simulink model "Energy_Storage_System"  (R2022b)
settings: Solver=FixedStepAuto  StartTime=0.0  StopTime=20000  FixedStep=1  RelTol=1e-3
model workspace (MAT data in the model file):
  C_space = 0.4
  Dilate = 0.1
  P0 = 100
  P_in_comp = 100
  T0 = 310
  T_coldwater_in = 293
  T_coldwater_out = 353
  T_in_comp = 300
  V_compress = 0.1
  V_storage = 310000
  Y_abhot = 1.295
  m0 = 320000
  rotor_speed = 80
settings Model: Creator=Crapon  LastModifiedBy=Crapon

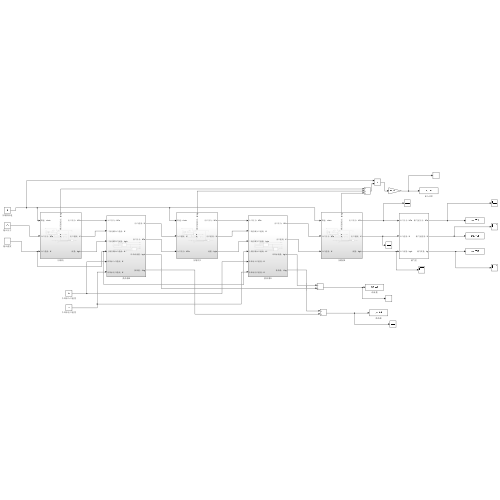
[thumbnail: Simulink's stored preview of the top-level diagram]
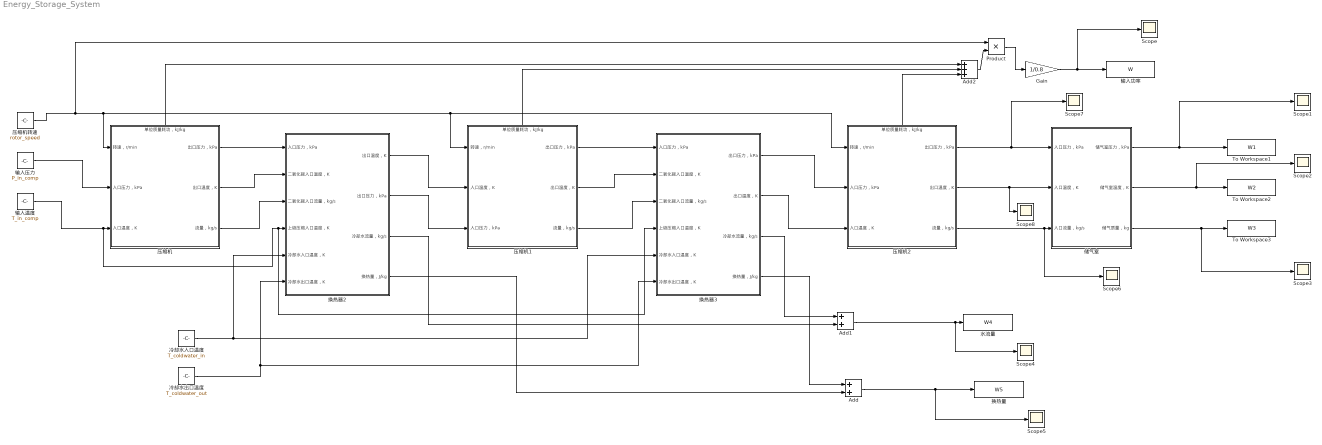
== system Energy_Storage_System ==
  Add : Sum
  Add1 : Sum
  Add2 : Sum  Inputs=+++
  Gain : Gain  Gain=1/0.8
  Product : Product
  Scope{,1..8} (9 alike) : Scope
  To Workspace1 : ToWorkspace  VariableName=W1  SaveFormat=Timeseries  SampleTime=-1
  To Workspace2 : ToWorkspace  VariableName=W2  SaveFormat=Timeseries  SampleTime=-1
  To Workspace3 : ToWorkspace  VariableName=W3  SaveFormat=Timeseries  SampleTime=-1
  储气室 : Subsystem
  冷却水入口温度 : Constant  Value=T_coldwater_in
  冷却水出口温度 : Constant  Value=T_coldwater_out
  压缩机 : Subsystem
      settings: PortSchema="{\"entries\":[{\"content\":{\"sides\":[{\"content\":{\"connectorIds\":[\"In1\",\"In2\",\"In3\"]},\"type\":\"ConnectorPlacement.EquallySpacedRectSide\",\"uuid\":\"17bf042e-cadd-48a6-8dfd-0be3cb7c0c8b\"},{\"content\":{\"connectorIds\":[\"Out1\",\"Out2\",\"Out3\"],\"side\":\"RIGHT\"},\"type\":\"ConnectorPlacement.EquallySpacedRectSide\",\"uuid\":\"9580532f-fe29-4788-9d7a-ca1c4a6711f8\"},{\"content\":{\"connectorIds\":[\"Out4\"],\"side\":\"TOP\"},\"type\":\"ConnectorPlacement.EquallySpacedRectSide\",\"uuid\":\"3a849305-9831-4dda-bb31-32b1caf0413e\"}]},\"type\":\"ConnectorPlacement.EquallySpacedConnector\",\"uuid\":\"fce5bf21-7d26-4726-80d8-4928c417d458\"}],\"packageUris\":[\"http://schema.mathworks.com/mf0/Connector/R2020b\"],\"version\":\"1.0\"}"
  压缩机1 : Subsystem
      settings: PortSchema="{\"entries\":[{\"content\":{\"sides\":[{\"content\":{\"connectorIds\":[\"In1\",\"In2\",\"In3\"]},\"type\":\"ConnectorPlacement.EquallySpacedRectSide\",\"uuid\":\"17bf042e-cadd-48a6-8dfd-0be3cb7c0c8b\"},{\"content\":{\"connectorIds\":[\"Out1\",\"Out2\",\"Out3\"],\"side\":\"RIGHT\"},\"type\":\"ConnectorPlacement.EquallySpacedRectSide\",\"uuid\":\"9580532f-fe29-4788-9d7a-ca1c4a6711f8\"},{\"content\":{\"connectorIds\":[\"Out4\"],\"side\":\"TOP\"},\"type\":\"ConnectorPlacement.EquallySpacedRectSide\",\"uuid\":\"3a849305-9831-4dda-bb31-32b1caf0413e\"}]},\"type\":\"ConnectorPlacement.EquallySpacedConnector\",\"uuid\":\"fce5bf21-7d26-4726-80d8-4928c417d458\"}],\"packageUris\":[\"http://schema.mathworks.com/mf0/Connector/R2020b\"],\"version\":\"1.0\"}"
  压缩机2 : Subsystem
      settings: PortSchema="{\"entries\":[{\"content\":{\"sides\":[{\"content\":{\"connectorIds\":[\"In1\",\"In2\",\"In3\"]},\"type\":\"ConnectorPlacement.EquallySpacedRectSide\",\"uuid\":\"17bf042e-cadd-48a6-8dfd-0be3cb7c0c8b\"},{\"content\":{\"connectorIds\":[\"Out1\",\"Out2\",\"Out3\"],\"side\":\"RIGHT\"},\"type\":\"ConnectorPlacement.EquallySpacedRectSide\",\"uuid\":\"9580532f-fe29-4788-9d7a-ca1c4a6711f8\"},{\"content\":{\"connectorIds\":[\"Out4\"],\"side\":\"TOP\"},\"type\":\"ConnectorPlacement.EquallySpacedRectSide\",\"uuid\":\"3a849305-9831-4dda-bb31-32b1caf0413e\"}]},\"type\":\"ConnectorPlacement.EquallySpacedConnector\",\"uuid\":\"fce5bf21-7d26-4726-80d8-4928c417d458\"}],\"packageUris\":[\"http://schema.mathworks.com/mf0/Connector/R2020b\"],\"version\":\"1.0\"}"
  压缩机转速 : Constant  Value=rotor_speed
  换热器2 : Subsystem
  换热器3 : Subsystem
  换热量 : ToWorkspace  VariableName=W5  SaveFormat=Timeseries  SampleTime=-1
  水流量 : ToWorkspace  VariableName=W4  SaveFormat=Timeseries  SampleTime=-1
  输入功率 : ToWorkspace  VariableName=W  SaveFormat=Timeseries  SampleTime=-1
  输入压力 : Constant  Value=P_in_comp
  输入温度 : Constant  Value=T_in_comp
  wires:
  压缩机/1(出口压力，kPa) -> 换热器2/1(入口压力，kPa)
  压缩机/2(出口温度，K) -> 换热器2/2(二氧化碳入口温度，K)
  压缩机/3(流量，kg/s) -> 换热器2/3(二氧化碳入口流量，kg/s)
  输入压力/1 -> 压缩机/2(入口压力，kPa)
  输入温度/1 -> 换热器3/4(上级压缩入口温度，K), 换热器2/4(上级压缩入口温度，K), 压缩机/3(入口温度，K)
  压缩机转速/1 -> Product/1, 压缩机/1(转速，r/min), 压缩机1/1(转速，r/min), 压缩机2/1(转速，r/min)
  压缩机1/1(出口压力，kPa) -> 换热器3/1(入口压力，kPa)
  压缩机1/2(出口温度，K) -> 换热器3/2(二氧化碳入口温度，K)
  压缩机1/3(流量，kg/s) -> 换热器3/3(二氧化碳入口流量，kg/s)
  换热器3/1(出口压力，kPa) -> 压缩机2/2(入口压力，kPa)
  换热器3/2(出口温度，K) -> 压缩机2/3(入口温度，K)
  压缩机2/1(出口压力，kPa) -> Scope7/1, 储气室/1(入口压力，kPa)
  压缩机2/2(出口温度，K) -> Scope8/1, 储气室/2(入口温度，K)
  压缩机2/3(流量，kg/s) -> Scope6/1, 储气室/3(入口流量，kg/s)
  换热器2/4(换热量，J/kg) -> Add/2
  换热器3/4(换热量，J/kg) -> Add/1
  换热器2/3(冷却水流量，kg/s) -> Add1/2
  换热器3/3(冷却水流量，kg/s) -> Add1/1
  压缩机/4(单位质量耗功，kJ/kg) -> Add2/1
  压缩机1/4(单位质量耗功，kJ/kg) -> Add2/2
  压缩机2/4(单位质量耗功，kJ/kg) -> Add2/3
  Gain/1 -> Scope/1, 输入功率/1
  储气室/1(储气室压力，kPa) -> To Workspace1/1, Scope1/1
  储气室/2(储气室温度，K) -> To Workspace2/1, Scope2/1
  储气室/3(储气质量，kg) -> Scope3/1, To Workspace3/1
  Add1/1 -> Scope4/1, 水流量/1
  Add/1 -> Scope5/1, 换热量/1
  冷却水入口温度/1 -> 换热器2/5(冷却水入口温度，K), 换热器3/5(冷却水入口温度，K)
  冷却水出口温度/1 -> 换热器3/6(冷却水出口温度，K), 换热器2/6(冷却水出口温度，K)
  换热器2/2(出口压力，kPa) -> 压缩机1/3(入口压力，kPa)
  换热器2/1(出口温度，K) -> 压缩机1/2(入口温度，K)
  Add2/1 -> Product/2
  Product/1 -> Gain/1

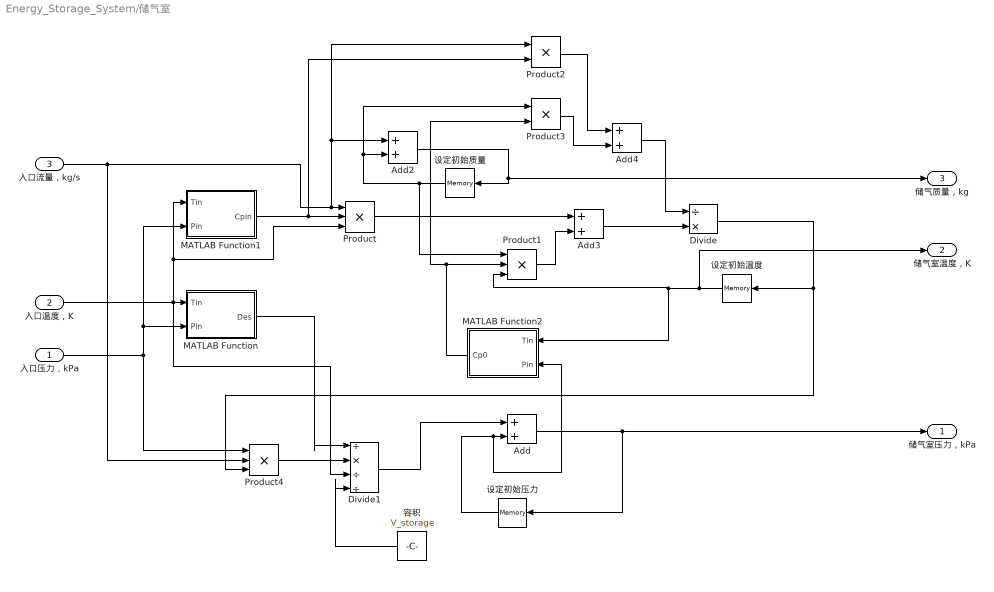
== system Energy_Storage_System/储气室 ==
  入口压力，kPa : Inport
  入口温度，K : Inport  Port=2
  入口流量，kg/s : Inport  Port=3
  Add{,2..4} (4 alike) : Sum
  Divide : Product  Inputs=/*
  Divide1 : Product  Inputs=/*//
  MATLAB Function : MATLAB Function  TreatAsAtomicUnit=on
  MATLAB Function1 : MATLAB Function  TreatAsAtomicUnit=on
  MATLAB Function2 : MATLAB Function  TreatAsAtomicUnit=on
  Product : Product  Inputs=3
  Product1 : Product  Inputs=3
  Product2 : Product
  Product3 : Product
  Product4 : Product  Inputs=3
  容积 : Constant  Value=V_storage
  设定初始压力 : Memory  InitialCondition=P0
  设定初始温度 : Memory  InitialCondition=T0
  设定初始质量 : Memory  InitialCondition=m0
  储气室压力，kPa : Outport
  储气室温度，K : Outport  Port=2
  储气质量，kg : Outport  Port=3
  wires:
  入口流量，kg/s/1 -> Product4/2, Product2/1, Add2/1, Product/1
  设定初始质量/1 -> Product1/1, Product3/1, Add2/2
  Product2/1 -> Add4/1
  MATLAB Function1/1(Cpin) -> Product/2, Product2/2
  Product4/1 -> Divide1/2
  MATLAB Function2/1(Cp0) -> Product1/2, Product3/2
  Divide1/1 -> Add/1
  入口温度，K/1 -> MATLAB Function1/1(Tin), Product/3, MATLAB Function/1(Tin), Divide1/3
  Product1/1 -> Add3/2
  Add/1 -> 储气室压力，kPa/1, 设定初始压力/1
  入口压力，kPa/1 -> Product4/1, MATLAB Function1/2(Pin), MATLAB Function/2(Pin)
  Add4/1 -> Divide/1
  设定初始压力/1 -> MATLAB Function2/2(Pin), Add/2
  容积/1 -> Divide1/4
  Product3/1 -> Add4/2
  MATLAB Function/1(Des) -> Divide1/1
  Add3/1 -> Divide/2
  Product/1 -> Add3/1
  Divide/1 -> Product4/3, 设定初始温度/1
  Add2/1 -> 设定初始质量/1, 储气质量，kg/1
  设定初始温度/1 -> 储气室温度，K/1, MATLAB Function2/1(Tin), Product1/3

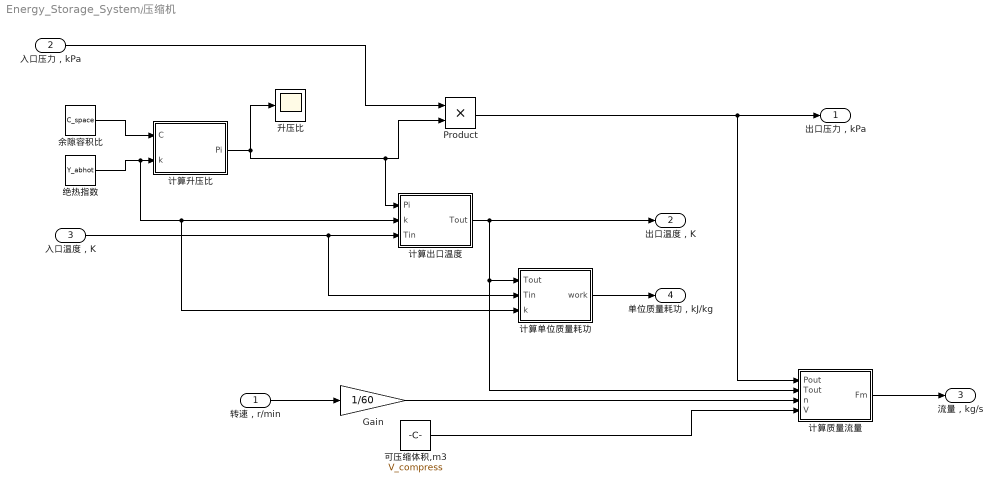
== system Energy_Storage_System/压缩机 ==
  转速，r/min : Inport
  入口压力，kPa : Inport  Port=2
  入口温度，K : Inport  Port=3
  Gain : Gain  Gain=1/60
  Product : Product
  余隙容积比 : Constant  Value=C_space
  升压比 : Scope
  可压缩体积,m3 : Constant  Value=V_compress
  绝热指数 : Constant  Value=Y_abhot
  计算出口温度 : MATLAB Function  TreatAsAtomicUnit=on
  计算升压比 : MATLAB Function  TreatAsAtomicUnit=on
  计算单位质量耗功 : MATLAB Function  TreatAsAtomicUnit=on
  计算质量流量 : MATLAB Function  TreatAsAtomicUnit=on
  出口压力，kPa : Outport
  出口温度，K : Outport  Port=2
  流量，kg/s : Outport  Port=3
  单位质量耗功，kJ/kg : Outport  Port=4
  wires:
  余隙容积比/1 -> 计算升压比/1(C)
  入口压力，kPa/1 -> Product/1
  绝热指数/1 -> 计算单位质量耗功/3(k), 计算出口温度/2(k), 计算升压比/2(k)
  Product/1 -> 计算质量流量/1(Pout), 出口压力，kPa/1
  计算单位质量耗功/1(work) -> 单位质量耗功，kJ/kg/1
  计算升压比/1(Pi) -> 计算出口温度/1(Pi), Product/2, 升压比/1
  入口温度，K/1 -> 计算单位质量耗功/2(Tin), 计算出口温度/3(Tin)
  计算出口温度/1(Tout) -> 出口温度，K/1, 计算质量流量/2(Tout), 计算单位质量耗功/1(Tout)
  计算质量流量/1(Fm) -> 流量，kg/s/1
  转速，r/min/1 -> Gain/1
  Gain/1 -> 计算质量流量/3(n)
  可压缩体积,m3/1 -> 计算质量流量/4(V)

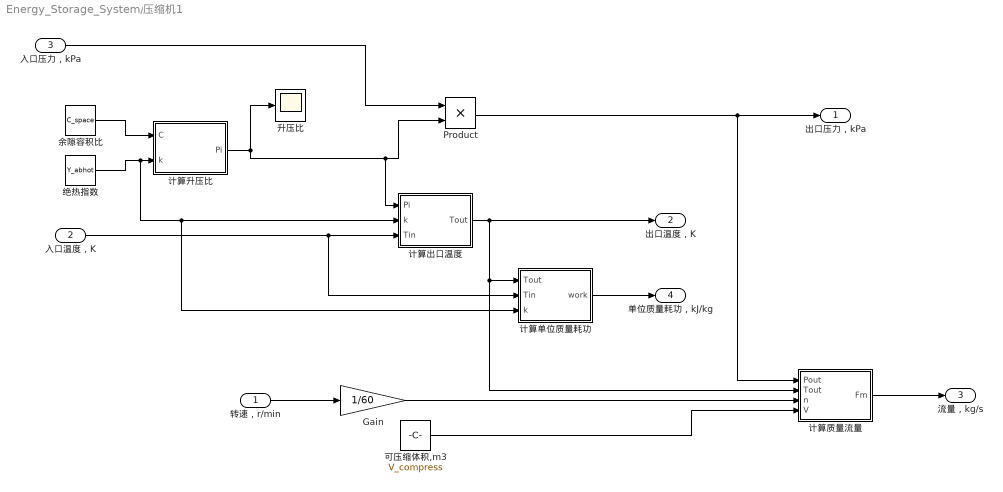
== system Energy_Storage_System/压缩机1 ==
  转速，r/min : Inport
  入口温度，K : Inport  Port=2
  入口压力，kPa : Inport  Port=3
  Gain : Gain  Gain=1/60
  Product : Product
  余隙容积比 : Constant  Value=C_space
  升压比 : Scope
  可压缩体积,m3 : Constant  Value=V_compress
  绝热指数 : Constant  Value=Y_abhot
  计算出口温度 : MATLAB Function  TreatAsAtomicUnit=on
  计算升压比 : MATLAB Function  TreatAsAtomicUnit=on
  计算单位质量耗功 : MATLAB Function  TreatAsAtomicUnit=on
  计算质量流量 : MATLAB Function  TreatAsAtomicUnit=on
  出口压力，kPa : Outport
  出口温度，K : Outport  Port=2
  流量，kg/s : Outport  Port=3
  单位质量耗功，kJ/kg : Outport  Port=4
  wires:
  可压缩体积,m3/1 -> 计算质量流量/4(V)
  Gain/1 -> 计算质量流量/3(n)
  转速，r/min/1 -> Gain/1
  计算质量流量/1(Fm) -> 流量，kg/s/1
  计算出口温度/1(Tout) -> 计算单位质量耗功/1(Tout), 计算质量流量/2(Tout), 出口温度，K/1
  入口温度，K/1 -> 计算出口温度/3(Tin), 计算单位质量耗功/2(Tin)
  计算升压比/1(Pi) -> 升压比/1, Product/2, 计算出口温度/1(Pi)
  计算单位质量耗功/1(work) -> 单位质量耗功，kJ/kg/1
  Product/1 -> 出口压力，kPa/1, 计算质量流量/1(Pout)
  绝热指数/1 -> 计算升压比/2(k), 计算出口温度/2(k), 计算单位质量耗功/3(k)
  入口压力，kPa/1 -> Product/1
  余隙容积比/1 -> 计算升压比/1(C)

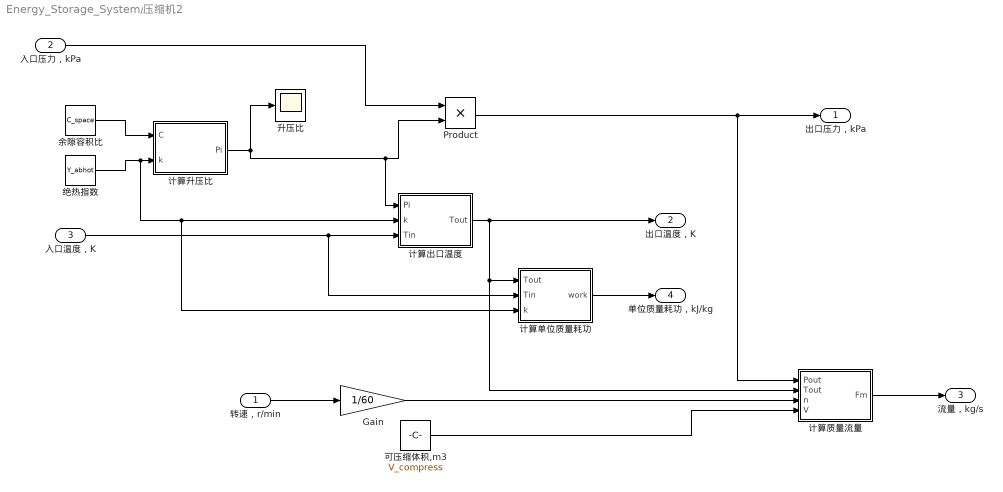
== system Energy_Storage_System/压缩机2 ==
  转速，r/min : Inport
  入口压力，kPa : Inport  Port=2
  入口温度，K : Inport  Port=3
  Gain : Gain  Gain=1/60
  Product : Product
  余隙容积比 : Constant  Value=C_space
  升压比 : Scope
  可压缩体积,m3 : Constant  Value=V_compress
  绝热指数 : Constant  Value=Y_abhot
  计算出口温度 : MATLAB Function  TreatAsAtomicUnit=on
  计算升压比 : MATLAB Function  TreatAsAtomicUnit=on
  计算单位质量耗功 : MATLAB Function  TreatAsAtomicUnit=on
  计算质量流量 : MATLAB Function  TreatAsAtomicUnit=on
  出口压力，kPa : Outport
  出口温度，K : Outport  Port=2
  流量，kg/s : Outport  Port=3
  单位质量耗功，kJ/kg : Outport  Port=4
  wires:
  余隙容积比/1 -> 计算升压比/1(C)
  入口压力，kPa/1 -> Product/1
  绝热指数/1 -> 计算单位质量耗功/3(k), 计算出口温度/2(k), 计算升压比/2(k)
  Product/1 -> 计算质量流量/1(Pout), 出口压力，kPa/1
  计算单位质量耗功/1(work) -> 单位质量耗功，kJ/kg/1
  计算升压比/1(Pi) -> 计算出口温度/1(Pi), Product/2, 升压比/1
  入口温度，K/1 -> 计算单位质量耗功/2(Tin), 计算出口温度/3(Tin)
  计算出口温度/1(Tout) -> 出口温度，K/1, 计算质量流量/2(Tout), 计算单位质量耗功/1(Tout)
  计算质量流量/1(Fm) -> 流量，kg/s/1
  转速，r/min/1 -> Gain/1
  Gain/1 -> 计算质量流量/3(n)
  可压缩体积,m3/1 -> 计算质量流量/4(V)

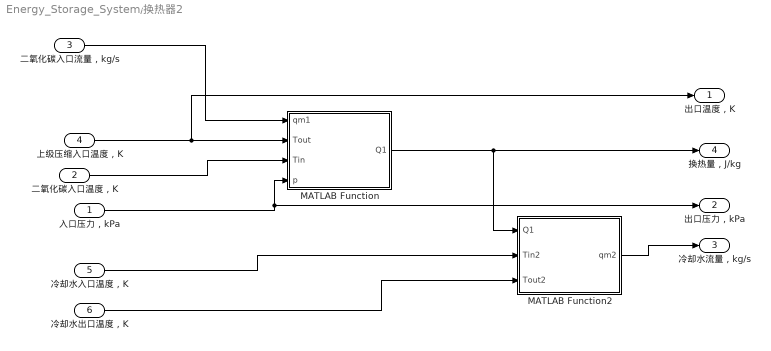
== system Energy_Storage_System/换热器2 ==
  入口压力，kPa : Inport
  二氧化碳入口温度，K : Inport  Port=2
  二氧化碳入口流量，kg/s : Inport  Port=3
  上级压缩入口温度，K : Inport  Port=4
  冷却水入口温度，K : Inport  Port=5
  冷却水出口温度，K : Inport  Port=6
  MATLAB Function : MATLAB Function  TreatAsAtomicUnit=on
  MATLAB Function2 : MATLAB Function  TreatAsAtomicUnit=on
  出口温度，K : Outport
  出口压力，kPa : Outport  Port=2
  冷却水流量，kg/s : Outport  Port=3
  换热量，J/kg : Outport  Port=4
  wires:
  入口压力，kPa/1 -> 出口压力，kPa/1, MATLAB Function/4(p)
  二氧化碳入口流量，kg/s/1 -> MATLAB Function/1(qm1)
  上级压缩入口温度，K/1 -> MATLAB Function/2(Tout), 出口温度，K/1
  二氧化碳入口温度，K/1 -> MATLAB Function/3(Tin)
  MATLAB Function2/1(qm2) -> 冷却水流量，kg/s/1
  冷却水入口温度，K/1 -> MATLAB Function2/2(Tin2)
  冷却水出口温度，K/1 -> MATLAB Function2/3(Tout2)
  MATLAB Function/1(Q1) -> MATLAB Function2/1(Q1), 换热量，J/kg/1

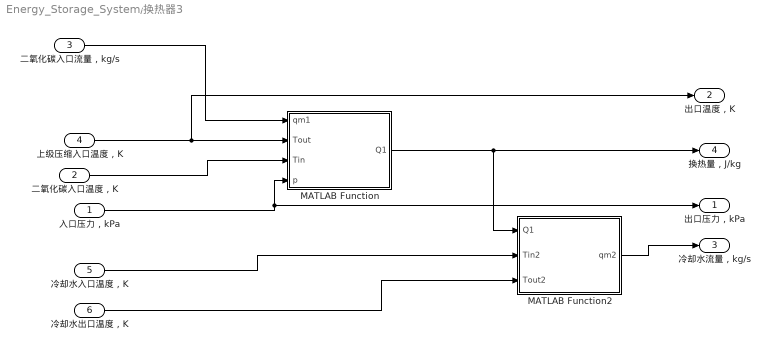
== system Energy_Storage_System/换热器3 ==
  入口压力，kPa : Inport
  二氧化碳入口温度，K : Inport  Port=2
  二氧化碳入口流量，kg/s : Inport  Port=3
  上级压缩入口温度，K : Inport  Port=4
  冷却水入口温度，K : Inport  Port=5
  冷却水出口温度，K : Inport  Port=6
  MATLAB Function : MATLAB Function  TreatAsAtomicUnit=on
  MATLAB Function2 : MATLAB Function  TreatAsAtomicUnit=on
  出口压力，kPa : Outport
  出口温度，K : Outport  Port=2
  冷却水流量，kg/s : Outport  Port=3
  换热量，J/kg : Outport  Port=4
  wires:
  MATLAB Function/1(Q1) -> 换热量，J/kg/1, MATLAB Function2/1(Q1)
  冷却水出口温度，K/1 -> MATLAB Function2/3(Tout2)
  冷却水入口温度，K/1 -> MATLAB Function2/2(Tin2)
  MATLAB Function2/1(qm2) -> 冷却水流量，kg/s/1
  二氧化碳入口温度，K/1 -> MATLAB Function/3(Tin)
  上级压缩入口温度，K/1 -> 出口温度，K/1, MATLAB Function/2(Tout)
  二氧化碳入口流量，kg/s/1 -> MATLAB Function/1(qm1)
  入口压力，kPa/1 -> MATLAB Function/4(p), 出口压力，kPa/1

== matlab function Energy_Storage_System/压缩机2/计算出口温度 ==
  data: Pi input; Tout output; k input; Tin input
function Tout= fcn(Pi, k, Tin)

Tout=Tin*(Pi)^((k-1)/k);

== matlab function Energy_Storage_System/储气室/MATLAB Function1 ==
  data: Tin input; Cpin output; Pin input
function Cpin = fcn(Tin,Pin)
coder.extrinsic('refpropm');
Cpin=zeros(1);
Cpin = refpropm('C','T',Tin,'P',Pin,'CO2');

== matlab function Energy_Storage_System/压缩机2/计算升压比 ==
  data: C input; Pi output; k input
function Pi = fcn(C, k)

Pi =(1+1/C)^k;

== matlab function Energy_Storage_System/压缩机2/计算单位质量耗功 ==
  data: Tout input; Tin input; k input; work output
function work= fcn(Tout,Tin,k)
Rg=0.189;
work=(k/(k-1))*Rg*(Tout-Tin);

== matlab function Energy_Storage_System/压缩机2/计算质量流量 ==
  data: Pout input; Tout input; n input; V input; Fm output
function Fm = fcn(Pout, Tout,n, V)
coder.extrinsic('refpropm');
a=zeros(1);
a=refpropm('D','T',Tout,'P',Pout,'CO2');
Fm = a*V*n;

== matlab function Energy_Storage_System/换热器2/MATLAB Function ==
  data: qm1 input; Tout input; Tin input; Q1 output; p input
function Q1 = fc(qm1,Tout,Tin,p)
coder.extrinsic('refpropm');
cp=zeros(1);
t=(Tin+Tout)/2;
cp=refpropm('C','T',t,'P',p,'CO2');
Q1= qm1*cp*(Tout-Tin);

== matlab function Energy_Storage_System/换热器2/MATLAB Function2 ==
  data: Q1 input; Tin2 input; Tout2 input; qm2 output
function qm2 = fcn(Q1,Tin2,Tout2)
coder.extrinsic('refpropm');
cp=zeros(1);
t=(Tin2+Tout2)/2;
cp=refpropm('C','T',t,'Q',0,'water');
qm2= Q1/(cp*(Tout2-Tin2));

== matlab function Energy_Storage_System/换热器3/MATLAB Function ==
  data: qm1 input; Tout input; Tin input; Q1 output; p input
function Q1 = fc(qm1,Tout,Tin,p)
coder.extrinsic('refpropm');
t=(Tin+Tout)/2;
cp=zeros(1);
cp=refpropm('C','T',t,'P',p,'CO2');
Q1= qm1*cp*(Tout-Tin);

== matlab function Energy_Storage_System/换热器3/MATLAB Function2 ==
  data: Q1 input; Tin2 input; Tout2 input; qm2 output
function qm2 = fcn(Q1,Tin2,Tout2)
coder.extrinsic('refpropm');
t=(Tin2+Tout2)/2;
cp=zeros(1);
cp=refpropm('C','T',t,'Q',0,'water');
qm2= Q1/(cp*(Tout2-Tin2));

== matlab function Energy_Storage_System/储气室/MATLAB Function ==
  data: Tin input; Des output; Pin input
function Des = fcn(Tin,Pin)
coder.extrinsic('refpropm');
Des=zeros(1);
Des = refpropm('D','T',Tin,'P',Pin,'CO2');

== matlab function Energy_Storage_System/储气室/MATLAB Function2 ==
  data: Tin input; Cp0 output; Pin input
function Cp0 = fcn(Tin,Pin)
coder.extrinsic('refpropm');
Cp0=zeros(1);
Cp0 = refpropm('C','T',Tin,'P',Pin,'CO2');

== matlab function Energy_Storage_System/压缩机/计算出口温度 ==
  data: Pi input; Tout output; k input; Tin input
function Tout= fcn(Pi, k, Tin)

Tout=Tin*(Pi)^((k-1)/k);

== matlab function Energy_Storage_System/压缩机/计算升压比 ==
  data: C input; Pi output; k input
function Pi = fcn(C, k)

Pi =(1+1/C)^k;

== matlab function Energy_Storage_System/压缩机/计算单位质量耗功 ==
  data: Tout input; Tin input; k input; work output
function work= fcn(Tout,Tin,k)
Rg=0.189;
work=(k/(k-1))*Rg*(Tout-Tin);

== matlab function Energy_Storage_System/压缩机/计算质量流量 ==
  data: Pout input; Tout input; n input; V input; Fm output
function Fm = fcn(Pout, Tout,n, V)
coder.extrinsic('refpropm');
a=zeros(1);
a=refpropm('D','T',Tout,'P',Pout,'CO2');
Fm = a*V*n;

== matlab function Energy_Storage_System/压缩机1/计算出口温度 ==
  data: Pi input; Tout output; k input; Tin input
function Tout= fcn(Pi, k, Tin)

Tout=Tin*(Pi)^((k-1)/k);

== matlab function Energy_Storage_System/压缩机1/计算升压比 ==
  data: C input; Pi output; k input
function Pi = fcn(C, k)

Pi =(1+1/C)^k;

== matlab function Energy_Storage_System/压缩机1/计算单位质量耗功 ==
  data: Tout input; Tin input; k input; work output
function work= fcn(Tout,Tin,k)
Rg=0.189;
work=(k/(k-1))*Rg*(Tout-Tin);

== matlab function Energy_Storage_System/压缩机1/计算质量流量 ==
  data: Pout input; Tout input; n input; V input; Fm output
function Fm = fcn(Pout, Tout,n, V)
coder.extrinsic('refpropm');
a=zeros(1);
a=refpropm('D','T',Tout,'P',Pout,'CO2');
Fm = a*V*n;
